simulink model "CuartoPunto"  (R2017b)
settings: Solver=VariableStepAuto  StartTime=0.0  StopTime=120  RelTol=1e-3
values from neighbouring files (symbols this model uses):
  g = -9.81    [Cuarto_Punto.m]
  h = 0.06    [Cuarto_Punto.m]
  jh = 0.0021    [Cuarto_Punto.m]
  jl = 0.0059    [Cuarto_Punto.m]
  kg = 70    [Cuarto_Punto.m]
  km = 0.00767    [Cuarto_Punto.m]
  ks = 1.61    [Cuarto_Punto.m]
  m = 0.403    [Cuarto_Punto.m]
  rm = 2.6    [Cuarto_Punto.m]
settings Model: Creator=franj  LastModifiedBy=franj

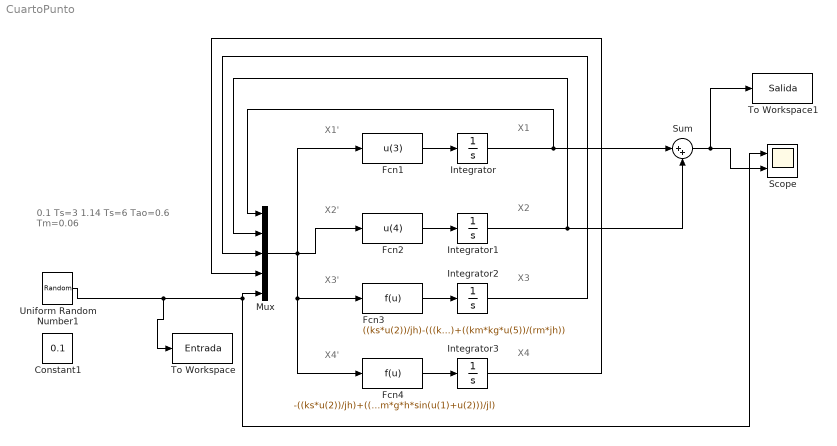
== system CuartoPunto ==
  note: X1
  note: X1'
  note: X2
  note: X2'
  note: X3
  note: X3'
  note: X4
  note: X4'
  note: 0.1 Ts=3
      | 1.14 Ts=6
      | Tao=0.6
      | Tm=0.06
  Constant1 : Constant  Value=0.1
  Fcn1 : Fcn  Expr=u(3)
  Fcn2 : Fcn  Expr=u(4)
  Fcn3 : Fcn  Expr=((ks*u(2))/jh)-(((km^2 )*(kg^2) *u(3))/(rm*jh))+((km*kg*u(5))/(rm*jh))
  Fcn4 : Fcn  Expr=-((ks*u(2))/jh)+(((km^2) *(kg^2) * u(3))/(rm*jh))-((km*kg*u(5))/(rm*jh))-((ks*u(2))/jl)+((m*g*h*sin(u(1)+u(2)))/jl)
  Integrator : Integrator
  Integrator1 : Integrator
  Integrator2 : Integrator  InitialCondition=0.1
  Integrator3 : Integrator
  Mux : Mux  Inputs=5
  Scope : Scope  NumInputPorts=2
  Sum : Sum  Inputs=|++
  To Workspace : ToWorkspace  VariableName=Entrada  SampleTime=0.06
  To Workspace1 : ToWorkspace  VariableName=Salida  SampleTime=0.06
  Uniform Random Number1 : UniformRandomNumber  Minimum=0.1  Maximum=1.14  SampleTime=6
  wires:
  Fcn1/1 -> Integrator/1
  Fcn2/1 -> Integrator1/1
  Fcn3/1 -> Integrator2/1
  Fcn4/1 -> Integrator3/1
  Mux/1 -> Fcn4/1, Fcn3/1, Fcn1/1, Fcn2/1
  Integrator/1 -> Mux/1, Sum/1
  Integrator1/1 -> Mux/2, Sum/2
  Integrator2/1 -> Mux/3
  Integrator3/1 -> Mux/4
  Uniform Random Number1/1 -> Mux/5, Scope/1, To Workspace/1
  Sum/1 -> To Workspace1/1, Scope/2
